simulink model "Prac03_2_2"  (R2015a)
settings: Solver=ode45  StartTime=0.0  StopTime=10.0  RelTol=1e-3
libraries: dspsigops x1
settings Model: Creator=Josemi  LastModifiedBy=Josemi

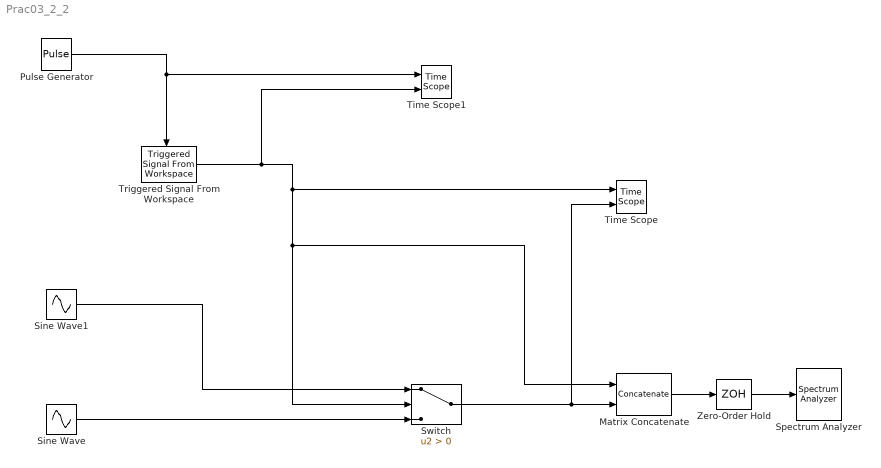
== system Prac03_2_2 ==
  Matrix Concatenate : Concatenate  Mode=Multidimensional array  ConcatenateDimension=2
  Pulse Generator : DiscretePulseGenerator  PulseType=Time based  Amplitude=0.5  Period=0.5  PulseWidth=50
  Sine Wave : Sin  Amplitude=0  Frequency=2*pi*10  SampleTime=0.0025
  Sine Wave1 : Sin  Amplitude=2  Frequency=2*pi*10  SampleTime=0.0025
  Spectrum Analyzer : SpectrumAnalyzer
  Switch : Switch  Criteria=u2 > Threshold  OutDataTypeStr=double
  Time Scope : TimeScope  DefaultConfigurationName=spbscopes.TimeScopeBlockCfg  NumInputPorts=2
  Time Scope1 : TimeScope  DefaultConfigurationName=spbscopes.TimeScopeBlockCfg  NumInputPorts=2
  Triggered Signal From Workspace : dspsigops/Triggered Signal From Workspace  Signal=[1 0 1 0 0 0 1 1 1 0 1 1 0 0 0]  TriggerType=Rising edge  ic=0  SamplesPerFrame=1  OutputAfterFinalValue=Setting to zero
  Zero-Order Hold : ZeroOrderHold  SampleTime=0.0025
  wires:
  Pulse Generator/1 -> Time Scope1/1, Triggered Signal From Workspace/Trigger
  Sine Wave1/1 -> Switch/1
  Sine Wave/1 -> Switch/3
  Triggered Signal From Workspace/1 -> Time Scope1/2, Switch/2, Matrix Concatenate/1, Time Scope/1
  Switch/1 -> Time Scope/2, Matrix Concatenate/2
  Matrix Concatenate/1 -> Zero-Order Hold/1
  Zero-Order Hold/1 -> Spectrum Analyzer/1
